simulink model "fuel_cell_model"  (R2022a)
settings: Solver=FixedStepAuto  StartTime=0.0  StopTime=220  FixedStep=0.01  RelTol=1e-3
settings Model: Creator=Learning  LastModifiedBy=Learning

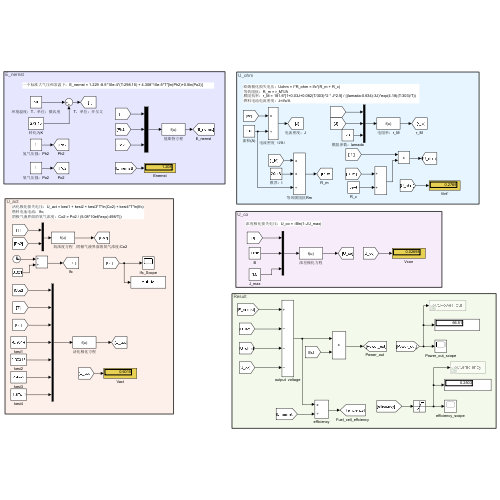
[thumbnail: Simulink's stored preview of the top-level diagram]
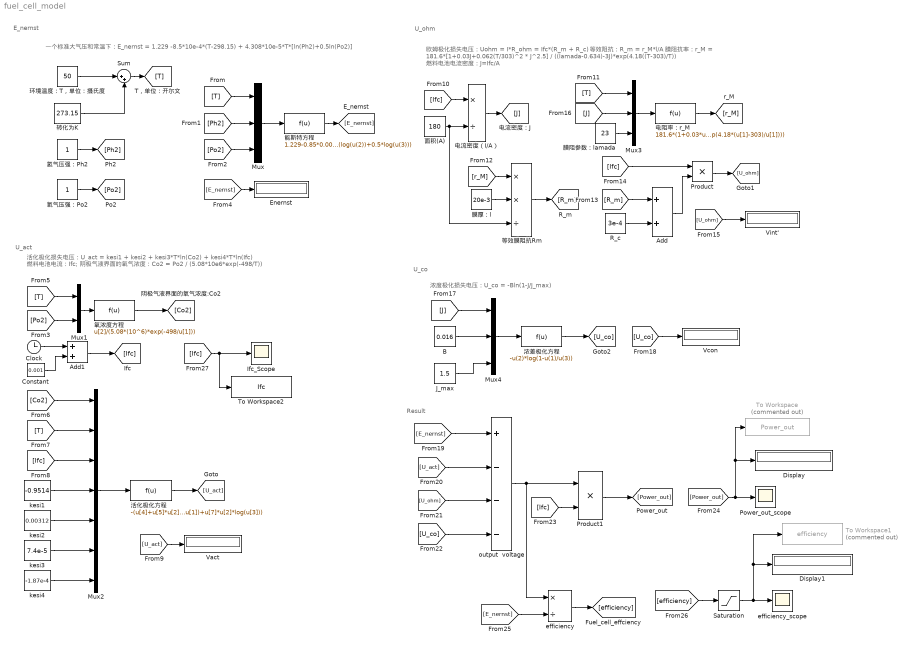
== system fuel_cell_model ==
  note: Result
  note: U_co
  note: 浓度极化损失电压：U_co = -Bln(1-J/J_max)
  note: U_ohm
  note: 欧姆极化损失电压：Uohm = I*R_ohm = Ifc*(R_m + R_c)
      | 等效阻抗：R_m = r_M*l/A
      | 膜阻抗率：r_M = 181.6*[1+0.03J+0.062(T/303)^2 * J^2.5] / ((lamada-0.634)-3J)*exp(4.18((T-303)/T))
      | 燃料电池电流密度：J=Ifc/A
  note: U_act
  note: 活化极化损失电压：U_act = kesi1 + kesi2 + kesi3*T*ln(Co2) + kesi4*T*ln(Ifc)
      | 燃料电池电流：Ifc;
      | 阴极气液界面的氧气浓度：Co2 = Po2 / (5.08*10e6*exp(-498/T))
  note: E_nernst
  note: 一个标准大气压和常温下：E_nernst = 1.229 -8.5*10e-4*(T-298.15) + 4.308*10e-5*T*[ln(Ph2)+0.5ln(Po2)]
  Add : Sum
  Add1 : Sum
  B : Constant  Value=0.016
  Clock : Clock
  Constant : Constant  Value=0.001
  Display : Display
  Display1 : Display
  Enernst : Display
      settings: Decimation=5
  Ifc_Scope : Scope
  J_max : Constant  Value=1.5
  Mux : Mux  Inputs=3
  Mux1 : Mux  Inputs=2
  Mux2 : Mux  Inputs=7
  Mux3 : Mux  Inputs=3
  Mux4 : Mux  Inputs=3
  Power_out_scope : Scope
  Product : Product
  Product1 : Product
  R_c : Constant  Value=3e-4
  Saturation : Saturate  UpperLimit=0.9  LowerLimit=0
  Sum : Sum  Inputs=|++
  To Workspace : ToWorkspace  Commented=on  VariableName=Power_out  SampleTime=-1
      settings: Save2DSignal=2-D array (concatenate along first dimension)
  To Workspace1 : ToWorkspace  Commented=on  VariableName=efficiency  SampleTime=-1
      settings: Save2DSignal=2-D array (concatenate along first dimension)
  To Workspace2 : ToWorkspace  VariableName=Ifc  SampleTime=-1
      settings: Save2DSignal=2-D array (concatenate along first dimension)
  Vact : Display
      settings: Decimation=5
  Vcon : Display
      settings: Decimation=5
  Vint' : Display
      settings: Decimation=5
  efficiency : Product  Inputs=*/  OutDataTypeStr=double
  efficiency_scope : Scope
  kesi1 : Constant  Value=-0.9514
  kesi2 : Constant  Value=0.00312
  kesi3 : Constant  Value=7.4e-5
  kesi4 : Constant  Value=-1.87e-4
  output  voltage : Sum  Inputs=+---  OutDataTypeStr=double
  氢气压强：Ph2 : Constant
  氧气压强：Po2 : Constant
  氧浓度方程 : Fcn  Expr=u[2]/(5.08*(10^6)*exp(-498/u[1]))
  活化极化方程 : Fcn  Expr=-(u[4]+u[5]*u[2]+u[6]*u[2]*log(u[1])+u[7]*u[2]*log(u[3]))
  浓差极化方程 : Fcn  Expr=-u(2)*log(1-u(1)/u(3))
  环境温度：T，单位：摄氏度 : Constant  Value=50
  电流密度（I/A） : Product  Inputs=*/  OutDataTypeStr=double
  电阻率：r_M : Fcn  Expr=181.6*(1+0.03*u[2]+0.062*((u[1]/303)^2)*(u[2]^2.5))/((u[3]-0.634-3*u[2])*(exp(4.18*(u[1]-303)/u[1])))
  等效膜阻抗Rm : Product  Inputs=**/  OutDataTypeStr=double
  能斯特方程 : Fcn  Expr=1.229-0.85*0.001*(u(1)-298.15)+4.3085*0.00001*u(1)*(log(u(2))+0.5*log(u(3)))
  膜厚：l : Constant  Value=20e-3
  膜阻参数：lamada : Constant  Value=23
  转化为K : Constant  Value=273.15
  面积(A) : Constant  Value=180
  wires:
  氢气压强：Ph2/1 -> [Ph2]
  氧气压强：Po2/1 -> [Po2]
  环境温度：T，单位：摄氏度/1 -> Sum/1
  Sum/1 -> [T]
  转化为K/1 -> Sum/2
  Mux/1 -> 能斯特方程/1
  [T] -> Mux/1
  [Ph2] -> Mux/2
  [Po2] -> Mux/3
  能斯特方程/1 -> [E_nernst]
  [E_nernst] -> Enernst/1
  Mux1/1 -> 氧浓度方程/1
  [T] -> Mux1/1
  [Po2] -> Mux1/2
  氧浓度方程/1 -> [Co2]
  kesi4/1 -> Mux2/7
  kesi3/1 -> Mux2/6
  kesi2/1 -> Mux2/5
  kesi1/1 -> Mux2/4
  [Ifc] -> Mux2/3
  [T] -> Mux2/2
  [Co2] -> Mux2/1
  [U_act] -> Vact/1
  Mux3/1 -> 电阻率：r_M/1
  [Ifc] -> 电流密度（I/A）/1
  面积(A)/1 -> 电流密度（I/A）/2, 等效膜阻抗Rm/3
  [T] -> Mux3/1
  膜阻参数：lamada/1 -> Mux3/3
  电阻率：r_M/1 -> [r_M]
  [r_M] -> 等效膜阻抗Rm/1
  膜厚：l/1 -> 等效膜阻抗Rm/2
  等效膜阻抗Rm/1 -> [R_m]
  [R_m] -> Add/1
  R_c/1 -> Add/2
  [Ifc] -> Product/1
  Add/1 -> Product/2
  Product/1 -> [U_ohm]
  [U_ohm] -> Vint'/1
  电流密度（I/A）/1 -> [J]
  [J] -> Mux3/2
  Mux4/1 -> 浓差极化方程/1
  [J] -> Mux4/1
  B/1 -> Mux4/2
  J_max/1 -> Mux4/3
  浓差极化方程/1 -> [U_co]
  [U_co] -> Vcon/1
  [E_nernst] -> output  voltage/1
  [U_act] -> output  voltage/2
  [U_ohm] -> output  voltage/3
  [U_co] -> output  voltage/4
  output  voltage/1 -> efficiency/1, Product1/1
  [Ifc] -> Product1/2
  Product1/1 -> [Power_out]
  [Power_out] -> To Workspace/1, Display/1, Power_out_scope/1
  [E_nernst] -> efficiency/2
  efficiency/1 -> [efficiency]
  [efficiency] -> Saturation/1
  Mux2/1 -> 活化极化方程/1
  活化极化方程/1 -> [U_act]
  [Ifc] -> To Workspace2/1, Ifc_Scope/1
  Clock/1 -> Add1/1
  Add1/1 -> [Ifc]
  Constant/1 -> Add1/2
  Saturation/1 -> efficiency_scope/1, To Workspace1/1, Display1/1
